simulink model "serialArduino"  (R2023b)
settings: Solver=VariableStepAuto  StartTime=0.0  StopTime=inf  RelTol=1e-3
undefined symbols (not defined in the file): LF
libraries: instrumentseriallib x9, etargetslib x3
settings Model: Creator=Bramantio  LastModifiedBy=Bramantio
settings OptimizationCC: ReuseModelBlockBuffer=off

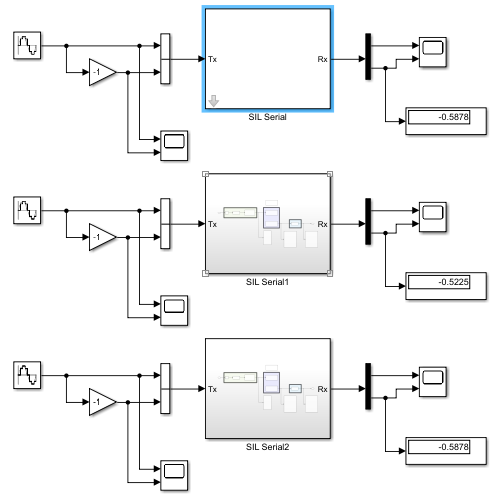
[thumbnail: Simulink's stored preview of the top-level diagram]
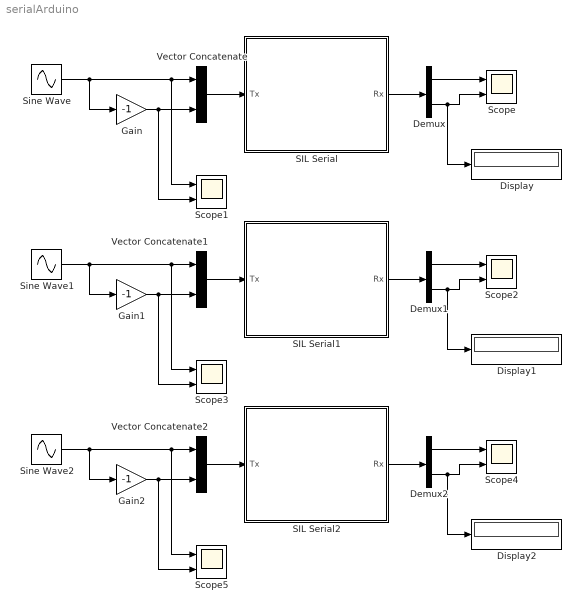
== system serialArduino ==
  Demux : Demux  Outputs=2
  Demux1 : Demux  Outputs=2
  Demux2 : Demux  Outputs=2
  Display : Display
  Display1 : Display
  Display2 : Display
  Gain : Gain  Gain=-1
  Gain1 : Gain  Gain=-1
  Gain2 : Gain  Gain=-1
  SIL Serial : Subsystem  mask{table=<empty>, Parameter2=0}
      mask TypeOptions table: <empty>
      mask DialogControl COM Prompt: COM
      mask DialogControl Container3 Prompt: BaudRate
  SIL Serial1 : Subsystem
  SIL Serial2 : Subsystem
  Scope{,1..5} (6 alike) : Scope  NumInputPorts=2
  Sine Wave : Sin  Frequency=2*pi*0.25  SampleTime=0.05
  Sine Wave1 : Sin  Frequency=2*pi*0.25  SampleTime=0.05
  Sine Wave2 : Sin  Frequency=2*pi*0.25  SampleTime=0.05
  Vector Concatenate : Concatenate
  Vector Concatenate1 : Concatenate
  Vector Concatenate2 : Concatenate
  wires:
  Gain/1 -> Scope1/2, Vector Concatenate/2
  Sine Wave/1 -> Scope1/1, Vector Concatenate/1, Gain/1
  Vector Concatenate/1 -> SIL Serial/1(Tx)
  SIL Serial/1(Rx) -> Demux/1
  Demux/1 -> Scope/1
  Demux/2 -> Display/1, Scope/2
  Demux1/2 -> Display1/1, Scope2/2
  Vector Concatenate1/1 -> SIL Serial1/1(Tx)
  SIL Serial1/1(Rx) -> Demux1/1
  Demux1/1 -> Scope2/1
  Sine Wave1/1 -> Scope3/1, Vector Concatenate1/1, Gain1/1
  Gain1/1 -> Scope3/2, Vector Concatenate1/2
  Gain2/1 -> Scope5/2, Vector Concatenate2/2
  SIL Serial2/1(Rx) -> Demux2/1
  Sine Wave2/1 -> Scope5/1, Vector Concatenate2/1, Gain2/1
  Vector Concatenate2/1 -> SIL Serial2/1(Tx)
  Demux2/1 -> Scope4/1
  Demux2/2 -> Display2/1, Scope4/2

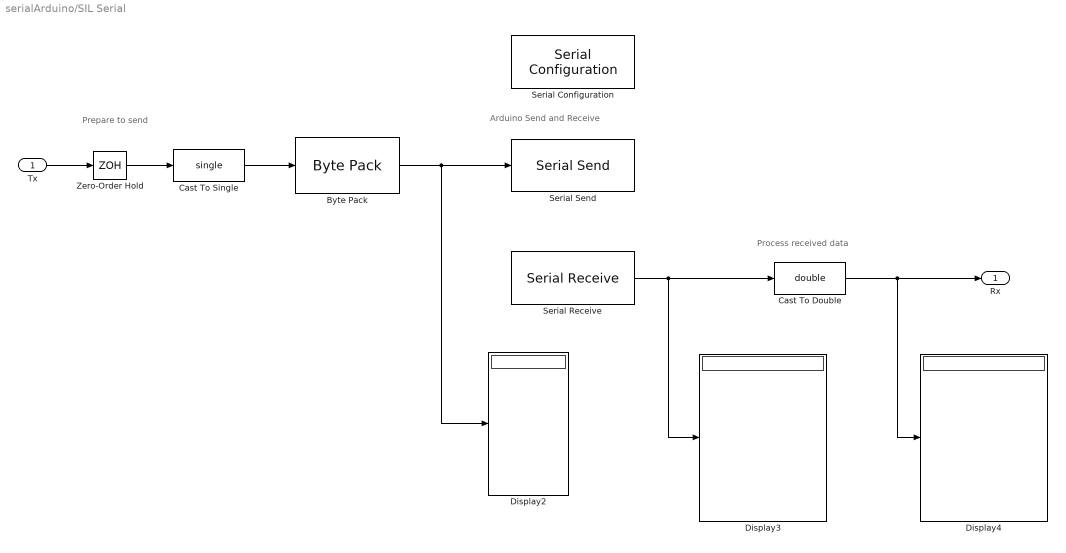
== system serialArduino/SIL Serial ==
  note: Prepare to send
  note: Arduino Send and Receive
  note: Process received data
  Tx : Inport
  Byte Pack : etargetslib/Byte Pack  datatypes={'single'}  byteAlign=4
  Cast To Double : DataTypeConversion  OutDataTypeStr=double  SaturateOnIntegerOverflow=off  RndMeth=Floor
  Cast To Single : DataTypeConversion  OutDataTypeStr=single  SaturateOnIntegerOverflow=off  RndMeth=Floor
  Display2 : Display
      settings: Format=hex (Stored Integer)
  Display3 : Display
  Display4 : Display
  Serial Configuration : instrumentseriallib/Serial Configuration  Priority=-200000  PortSel=COM7  Port=COM7  ComPort=COM7  BaudRate=115200  DataBits=8  Parity=none  StopBits=1  ByteOrder=little-endian  FlowControl=none  Timeout=10  SimulateUsing=Interpreted execution  BlockInModel=on  aMode=1
  Serial Receive : instrumentseriallib/Serial Receive  Priority=1  PortSel=COM7  Port=COM7  ComPort=COM7  DataType=single  SaveDataType=uint8  ToggleHeader=on  Header=[ 65 ]  ToggleTerminator=on  Terminator=LF ('\n')  CustomTerminator=[]  InputFormat=Column major  ToggleDataSize=on  DataSize=[1 2]  EnableBlockingMode=on  ActionDataUnavailable=Output last received value  ActionWhenDataUnavailable=Output last received value  CustomValue=0  SampleTime=0.05  SimulateUsing=Interpreted execution  BlockInModel=on  aMode=1
  Serial Send : instrumentseriallib/Serial Send  Priority=1  PortSel=COM7  Port=COM7  ComPort=COM7  Header=[]  Terminator=LF ('\n')  CustomTerminator=[]  EnableBlockingMode=on  SimulateUsing=Interpreted execution  BlockInModel=on  aMode=1
  Zero-Order Hold : ZeroOrderHold  SampleTime=0.05
  Rx : Outport
  wires:
  Tx/1 -> Zero-Order Hold/1
  Serial Receive/1 -> Display3/1, Cast To Double/1
  Zero-Order Hold/1 -> Cast To Single/1
  Byte Pack/1 -> Display2/1, Serial Send/1
  Cast To Double/1 -> Display4/1, Rx/1
  Cast To Single/1 -> Byte Pack/1

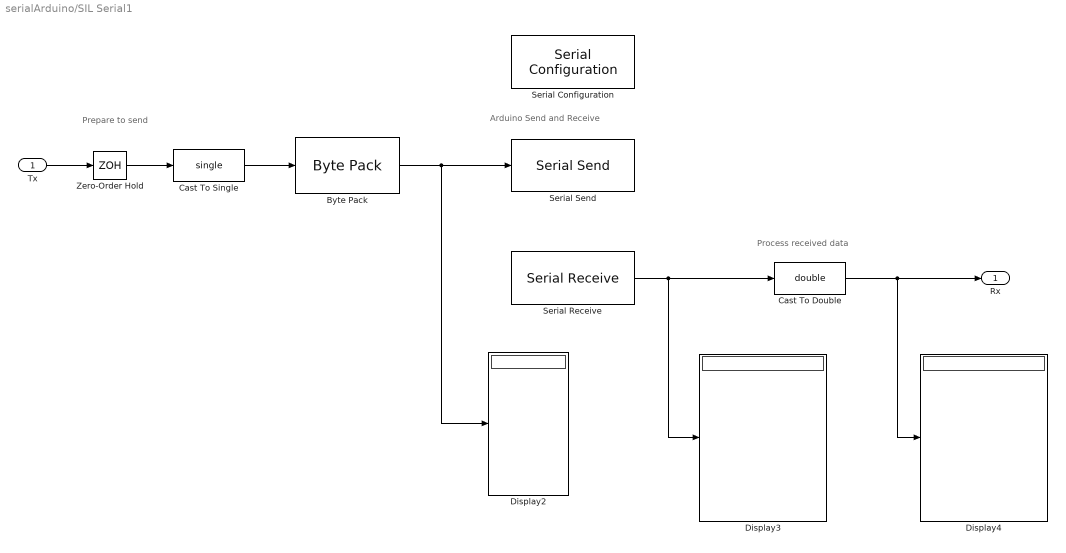
== system serialArduino/SIL Serial1 ==
  note: Prepare to send
  note: Arduino Send and Receive
  note: Process received data
  Tx : Inport
  Byte Pack : etargetslib/Byte Pack  datatypes={'single'}  byteAlign=4
  Cast To Double : DataTypeConversion  OutDataTypeStr=double  SaturateOnIntegerOverflow=off  RndMeth=Floor
  Cast To Single : DataTypeConversion  OutDataTypeStr=single  SaturateOnIntegerOverflow=off  RndMeth=Floor
  Display2 : Display
      settings: Format=hex (Stored Integer)
  Display3 : Display
  Display4 : Display
  Serial Configuration : instrumentseriallib/Serial Configuration  Priority=-200000  PortSel=COM8  Port=COM8  ComPort=COM8  BaudRate=115200  DataBits=8  Parity=none  StopBits=1  ByteOrder=little-endian  FlowControl=none  Timeout=10  SimulateUsing=Interpreted execution  BlockInModel=on  aMode=1
  Serial Receive : instrumentseriallib/Serial Receive  Priority=1  PortSel=COM8  Port=COM8  ComPort=COM8  DataType=single  SaveDataType=uint8  ToggleHeader=on  Header=[ 65 ]  ToggleTerminator=on  Terminator=LF ('\n')  CustomTerminator=[]  InputFormat=Column major  ToggleDataSize=on  DataSize=[1 2]  EnableBlockingMode=on  ActionDataUnavailable=Output last received value  ActionWhenDataUnavailable=Output last received value  CustomValue=0  SampleTime=0.05  SimulateUsing=Interpreted execution  BlockInModel=on  aMode=1
  Serial Send : instrumentseriallib/Serial Send  Priority=1  PortSel=COM8  Port=COM8  ComPort=COM8  Header=[]  Terminator=LF ('\n')  CustomTerminator=[]  EnableBlockingMode=on  SimulateUsing=Interpreted execution  BlockInModel=on  aMode=1
  Zero-Order Hold : ZeroOrderHold  SampleTime=0.05
  Rx : Outport
  wires:
  Tx/1 -> Zero-Order Hold/1
  Serial Receive/1 -> Display3/1, Cast To Double/1
  Zero-Order Hold/1 -> Cast To Single/1
  Byte Pack/1 -> Display2/1, Serial Send/1
  Cast To Double/1 -> Display4/1, Rx/1
  Cast To Single/1 -> Byte Pack/1

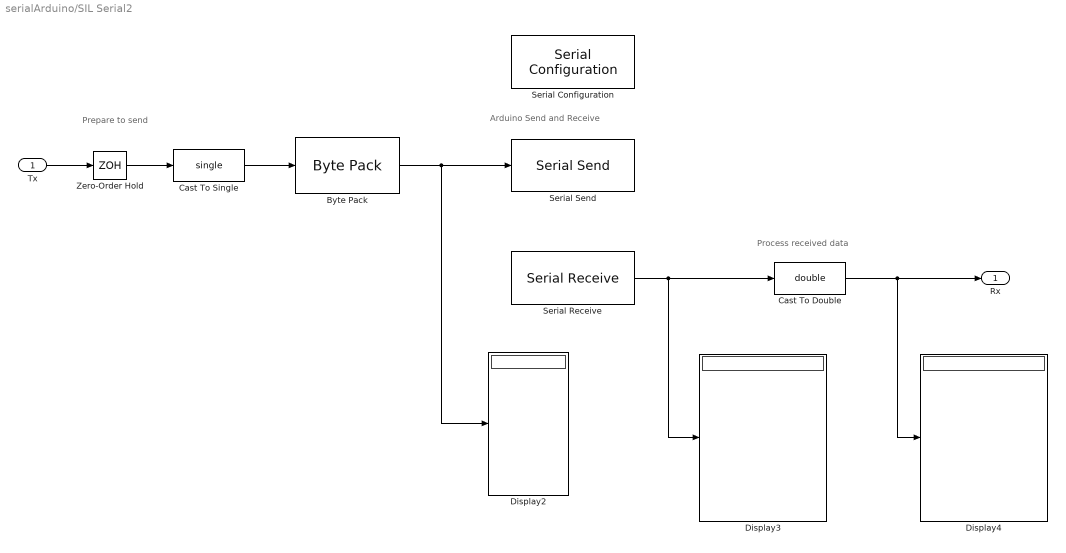
== system serialArduino/SIL Serial2 ==
  note: Prepare to send
  note: Arduino Send and Receive
  note: Process received data
  Tx : Inport
  Byte Pack : etargetslib/Byte Pack  datatypes={'single'}  byteAlign=4
  Cast To Double : DataTypeConversion  OutDataTypeStr=double  SaturateOnIntegerOverflow=off  RndMeth=Floor
  Cast To Single : DataTypeConversion  OutDataTypeStr=single  SaturateOnIntegerOverflow=off  RndMeth=Floor
  Display2 : Display
      settings: Format=hex (Stored Integer)
  Display3 : Display
  Display4 : Display
  Serial Configuration : instrumentseriallib/Serial Configuration  Priority=-200000  PortSel=COM9  Port=COM9  ComPort=COM9  BaudRate=115200  DataBits=8  Parity=none  StopBits=1  ByteOrder=little-endian  FlowControl=none  Timeout=10  SimulateUsing=Interpreted execution  BlockInModel=on  aMode=1
  Serial Receive : instrumentseriallib/Serial Receive  Priority=1  PortSel=COM9  Port=COM9  ComPort=COM9  DataType=single  SaveDataType=uint8  ToggleHeader=on  Header=[ 65 ]  ToggleTerminator=on  Terminator=LF ('\n')  CustomTerminator=[]  InputFormat=Column major  ToggleDataSize=on  DataSize=[1 2]  EnableBlockingMode=on  ActionDataUnavailable=Output last received value  ActionWhenDataUnavailable=Output last received value  CustomValue=0  SampleTime=0.05  SimulateUsing=Interpreted execution  BlockInModel=on  aMode=1
  Serial Send : instrumentseriallib/Serial Send  Priority=1  PortSel=COM9  Port=COM9  ComPort=COM9  Header=[]  Terminator=LF ('\n')  CustomTerminator=[]  EnableBlockingMode=on  SimulateUsing=Interpreted execution  BlockInModel=on  aMode=1
  Zero-Order Hold : ZeroOrderHold  SampleTime=0.05
  Rx : Outport
  wires:
  Tx/1 -> Zero-Order Hold/1
  Serial Receive/1 -> Display3/1, Cast To Double/1
  Zero-Order Hold/1 -> Cast To Single/1
  Byte Pack/1 -> Display2/1, Serial Send/1
  Cast To Double/1 -> Display4/1, Rx/1
  Cast To Single/1 -> Byte Pack/1
